simulink model "Problem1"  (R2016a)
settings: Solver=VariableStepAuto  StartTime=0.0  StopTime=20  RelTol=1e-3
settings Model: Creator=acala  LastModifiedBy=acala

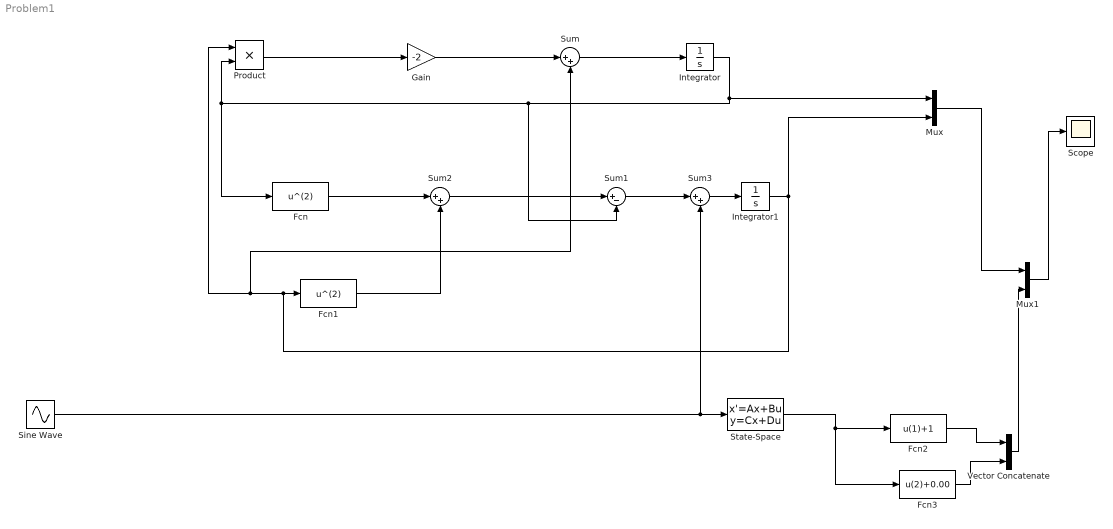
== system Problem1 ==
  Fcn : Fcn  Expr=u^(2)
  Fcn1 : Fcn  Expr=u^(2)
  Fcn2 : Fcn  Expr=u(1)+1
  Fcn3 : Fcn  Expr=u(2)+0.00
  Gain : Gain  Gain=-2
  Integrator : Integrator  InitialCondition=1
  Integrator1 : Integrator
  Mux : Mux  Inputs=2
  Mux1 : Mux  Inputs=2
  Product : Product
  Scope : Scope
  Sine Wave : Sin  Amplitude=0.01  SampleTime=0
  State-Space : StateSpace  A=[0,-1;1,0]  B=[0;1]  C=[1,0;0,1]  D=[0;0]  X0=[0;0]
  Sum : Sum  Inputs=|++
  Sum1 : Sum  Inputs=|+-
  Sum2 : Sum  Inputs=|++
  Sum3 : Sum  Inputs=|++
  Vector Concatenate : Concatenate
  wires:
  Sum/1 -> Integrator/1
  Gain/1 -> Sum/1
  Product/1 -> Gain/1
  Sum1/1 -> Sum3/1
  Sum2/1 -> Sum1/1
  Fcn/1 -> Sum2/1
  Fcn1/1 -> Sum2/2
  Integrator/1 -> Mux/1, Fcn/1, Product/2, Sum1/2
  Sine Wave/1 -> State-Space/1, Sum3/2
  Sum3/1 -> Integrator1/1
  Integrator1/1 -> Fcn1/1, Sum/2, Product/1, Mux/2
  Mux1/1 -> Scope/1
  State-Space/1 -> Fcn3/1, Fcn2/1
  Fcn2/1 -> Vector Concatenate/1
  Fcn3/1 -> Vector Concatenate/2
  Vector Concatenate/1 -> Mux1/2
  Mux/1 -> Mux1/1
